simulink model "PTTransmCU"  (Simulink 10.3)
settings: Solver=ode45  StartTime=0.0  StopTime=inf  RelTol=1e-3  EnableMultiTasking=on
libraries: simulink x2, CarMaker4SL x1
(part 3 of 4)

== system PTTransmCU/CarMaker/IPG Vehicle/PowerTrain/TCU Example/PTTransmCU_In/CreateBus TCU ClutchIn5 ==
  In : Inport
  BusCreator : BusCreator  Inputs=7
  Demux : Demux  Outputs=7
      settings: DisplayOption=none
  Out : Outport  VectorParamsAs1DForOutWhenUnconnected=off
  wires:
  Demux/7 -> BusCreator/7  "TCU ClutchIn5 i_TrqIn2Out"
  Demux/6 -> BusCreator/6  "TCU ClutchIn5 Trq_out_trg"
  Demux/5 -> BusCreator/5  "TCU ClutchIn5 Trq_out"
  Demux/4 -> BusCreator/4  "TCU ClutchIn5 Trq_in"
  Demux/3 -> BusCreator/3  "TCU ClutchIn5 rotv_out_trg"
  Demux/2 -> BusCreator/2  "TCU ClutchIn5 rotv_out"
  Demux/1 -> BusCreator/1  "TCU ClutchIn5 rotv_in"
  BusCreator/1 -> Out/1
  In/1 -> Demux/1

== system PTTransmCU/CarMaker/IPG Vehicle/PowerTrain/TCU Example/PTTransmCU_In/CreateBus TCU ClutchIn6 ==
  In : Inport
  BusCreator : BusCreator  Inputs=7
  Demux : Demux  Outputs=7
      settings: DisplayOption=none
  Out : Outport  VectorParamsAs1DForOutWhenUnconnected=off
  wires:
  Demux/7 -> BusCreator/7  "TCU ClutchIn6 i_TrqIn2Out"
  Demux/6 -> BusCreator/6  "TCU ClutchIn6 Trq_out_trg"
  Demux/5 -> BusCreator/5  "TCU ClutchIn6 Trq_out"
  Demux/4 -> BusCreator/4  "TCU ClutchIn6 Trq_in"
  Demux/3 -> BusCreator/3  "TCU ClutchIn6 rotv_out_trg"
  Demux/2 -> BusCreator/2  "TCU ClutchIn6 rotv_out"
  Demux/1 -> BusCreator/1  "TCU ClutchIn6 rotv_in"
  BusCreator/1 -> Out/1
  In/1 -> Demux/1

== system PTTransmCU/CarMaker/IPG Vehicle/PowerTrain/TCU Example/PTTransmCU_In/CreateBus TCU ClutchIn7 ==
  In : Inport
  BusCreator : BusCreator  Inputs=7
  Demux : Demux  Outputs=7
      settings: DisplayOption=none
  Out : Outport  VectorParamsAs1DForOutWhenUnconnected=off
  wires:
  Demux/7 -> BusCreator/7  "TCU ClutchIn7 i_TrqIn2Out"
  Demux/6 -> BusCreator/6  "TCU ClutchIn7 Trq_out_trg"
  Demux/5 -> BusCreator/5  "TCU ClutchIn7 Trq_out"
  Demux/4 -> BusCreator/4  "TCU ClutchIn7 Trq_in"
  Demux/3 -> BusCreator/3  "TCU ClutchIn7 rotv_out_trg"
  Demux/2 -> BusCreator/2  "TCU ClutchIn7 rotv_out"
  Demux/1 -> BusCreator/1  "TCU ClutchIn7 rotv_in"
  BusCreator/1 -> Out/1
  In/1 -> Demux/1

== system PTTransmCU/CarMaker/IPG Vehicle/PowerTrain/TCU Example/PTTransmCU_In/CreateBus TCU ClutchIn8 ==
  In : Inport
  BusCreator : BusCreator  Inputs=7
  Demux : Demux  Outputs=7
      settings: DisplayOption=none
  Out : Outport  VectorParamsAs1DForOutWhenUnconnected=off
  wires:
  Demux/7 -> BusCreator/7  "TCU ClutchIn8 i_TrqIn2Out"
  Demux/6 -> BusCreator/6  "TCU ClutchIn8 Trq_out_trg"
  Demux/5 -> BusCreator/5  "TCU ClutchIn8 Trq_out"
  Demux/4 -> BusCreator/4  "TCU ClutchIn8 Trq_in"
  Demux/3 -> BusCreator/3  "TCU ClutchIn8 rotv_out_trg"
  Demux/2 -> BusCreator/2  "TCU ClutchIn8 rotv_out"
  Demux/1 -> BusCreator/1  "TCU ClutchIn8 rotv_in"
  BusCreator/1 -> Out/1
  In/1 -> Demux/1

== system PTTransmCU/CarMaker/IPG Vehicle/PowerTrain/TCU Example/PTTransmCU_In/CreateBus TCU ClutchIn9 ==
  In : Inport
  BusCreator : BusCreator  Inputs=7
  Demux : Demux  Outputs=7
      settings: DisplayOption=none
  Out : Outport  VectorParamsAs1DForOutWhenUnconnected=off
  wires:
  Demux/7 -> BusCreator/7  "TCU ClutchIn9 i_TrqIn2Out"
  Demux/6 -> BusCreator/6  "TCU ClutchIn9 Trq_out_trg"
  Demux/5 -> BusCreator/5  "TCU ClutchIn9 Trq_out"
  Demux/4 -> BusCreator/4  "TCU ClutchIn9 Trq_in"
  Demux/3 -> BusCreator/3  "TCU ClutchIn9 rotv_out_trg"
  Demux/2 -> BusCreator/2  "TCU ClutchIn9 rotv_out"
  Demux/1 -> BusCreator/1  "TCU ClutchIn9 rotv_in"
  BusCreator/1 -> Out/1
  In/1 -> Demux/1

== system PTTransmCU/CarMaker/IPG Vehicle/PowerTrain/TCU Example/PTTransmCU_In/CreateBus TCU ClutchOut0 ==
  In : Inport
  BusCreator : BusCreator  Inputs=1
  Demux : Demux  Outputs=1
      settings: DisplayOption=none
  Out : Outport  VectorParamsAs1DForOutWhenUnconnected=off
  wires:
  Demux/1 -> BusCreator/1  "TCU ClutchOut0 Pos"
  BusCreator/1 -> Out/1
  In/1 -> Demux/1

== system PTTransmCU/CarMaker/IPG Vehicle/PowerTrain/TCU Example/PTTransmCU_In/CreateBus TCU ClutchOut1 ==
  In : Inport
  BusCreator : BusCreator  Inputs=1
  Demux : Demux  Outputs=1
      settings: DisplayOption=none
  Out : Outport  VectorParamsAs1DForOutWhenUnconnected=off
  wires:
  Demux/1 -> BusCreator/1  "TCU ClutchOut1 Pos"
  BusCreator/1 -> Out/1
  In/1 -> Demux/1

== system PTTransmCU/CarMaker/IPG Vehicle/PowerTrain/TCU Example/PTTransmCU_In/CreateBus TCU ClutchOut10 ==
  In : Inport
  BusCreator : BusCreator  Inputs=1
  Demux : Demux  Outputs=1
      settings: DisplayOption=none
  Out : Outport  VectorParamsAs1DForOutWhenUnconnected=off
  wires:
  Demux/1 -> BusCreator/1  "TCU ClutchOut10 Pos"
  BusCreator/1 -> Out/1
  In/1 -> Demux/1

== system PTTransmCU/CarMaker/IPG Vehicle/PowerTrain/TCU Example/PTTransmCU_In/CreateBus TCU ClutchOut11 ==
  In : Inport
  BusCreator : BusCreator  Inputs=1
  Demux : Demux  Outputs=1
      settings: DisplayOption=none
  Out : Outport  VectorParamsAs1DForOutWhenUnconnected=off
  wires:
  Demux/1 -> BusCreator/1  "TCU ClutchOut11 Pos"
  BusCreator/1 -> Out/1
  In/1 -> Demux/1

== system PTTransmCU/CarMaker/IPG Vehicle/PowerTrain/TCU Example/PTTransmCU_In/CreateBus TCU ClutchOut2 ==
  In : Inport
  BusCreator : BusCreator  Inputs=1
  Demux : Demux  Outputs=1
      settings: DisplayOption=none
  Out : Outport  VectorParamsAs1DForOutWhenUnconnected=off
  wires:
  Demux/1 -> BusCreator/1  "TCU ClutchOut2 Pos"
  BusCreator/1 -> Out/1
  In/1 -> Demux/1

== system PTTransmCU/CarMaker/IPG Vehicle/PowerTrain/TCU Example/PTTransmCU_In/CreateBus TCU ClutchOut3 ==
  In : Inport
  BusCreator : BusCreator  Inputs=1
  Demux : Demux  Outputs=1
      settings: DisplayOption=none
  Out : Outport  VectorParamsAs1DForOutWhenUnconnected=off
  wires:
  Demux/1 -> BusCreator/1  "TCU ClutchOut3 Pos"
  BusCreator/1 -> Out/1
  In/1 -> Demux/1

== system PTTransmCU/CarMaker/IPG Vehicle/PowerTrain/TCU Example/PTTransmCU_In/CreateBus TCU ClutchOut4 ==
  In : Inport
  BusCreator : BusCreator  Inputs=1
  Demux : Demux  Outputs=1
      settings: DisplayOption=none
  Out : Outport  VectorParamsAs1DForOutWhenUnconnected=off
  wires:
  Demux/1 -> BusCreator/1  "TCU ClutchOut4 Pos"
  BusCreator/1 -> Out/1
  In/1 -> Demux/1

== system PTTransmCU/CarMaker/IPG Vehicle/PowerTrain/TCU Example/PTTransmCU_In/CreateBus TCU ClutchOut5 ==
  In : Inport
  BusCreator : BusCreator  Inputs=1
  Demux : Demux  Outputs=1
      settings: DisplayOption=none
  Out : Outport  VectorParamsAs1DForOutWhenUnconnected=off
  wires:
  Demux/1 -> BusCreator/1  "TCU ClutchOut5 Pos"
  BusCreator/1 -> Out/1
  In/1 -> Demux/1

== system PTTransmCU/CarMaker/IPG Vehicle/PowerTrain/TCU Example/PTTransmCU_In/CreateBus TCU ClutchOut6 ==
  In : Inport
  BusCreator : BusCreator  Inputs=1
  Demux : Demux  Outputs=1
      settings: DisplayOption=none
  Out : Outport  VectorParamsAs1DForOutWhenUnconnected=off
  wires:
  Demux/1 -> BusCreator/1  "TCU ClutchOut6 Pos"
  BusCreator/1 -> Out/1
  In/1 -> Demux/1

== system PTTransmCU/CarMaker/IPG Vehicle/PowerTrain/TCU Example/PTTransmCU_In/CreateBus TCU ClutchOut7 ==
  In : Inport
  BusCreator : BusCreator  Inputs=1
  Demux : Demux  Outputs=1
      settings: DisplayOption=none
  Out : Outport  VectorParamsAs1DForOutWhenUnconnected=off
  wires:
  Demux/1 -> BusCreator/1  "TCU ClutchOut7 Pos"
  BusCreator/1 -> Out/1
  In/1 -> Demux/1

== system PTTransmCU/CarMaker/IPG Vehicle/PowerTrain/TCU Example/PTTransmCU_In/CreateBus TCU ClutchOut8 ==
  In : Inport
  BusCreator : BusCreator  Inputs=1
  Demux : Demux  Outputs=1
      settings: DisplayOption=none
  Out : Outport  VectorParamsAs1DForOutWhenUnconnected=off
  wires:
  Demux/1 -> BusCreator/1  "TCU ClutchOut8 Pos"
  BusCreator/1 -> Out/1
  In/1 -> Demux/1

== system PTTransmCU/CarMaker/IPG Vehicle/PowerTrain/TCU Example/PTTransmCU_In/CreateBus TCU ClutchOut9 ==
  In : Inport
  BusCreator : BusCreator  Inputs=1
  Demux : Demux  Outputs=1
      settings: DisplayOption=none
  Out : Outport  VectorParamsAs1DForOutWhenUnconnected=off
  wires:
  Demux/1 -> BusCreator/1  "TCU ClutchOut9 Pos"
  BusCreator/1 -> Out/1
  In/1 -> Demux/1

== system PTTransmCU/CarMaker/IPG Vehicle/PowerTrain/TCU Example/PTTransmCU_In/CreateBus TCU GearboxIn0 ==
  In : Inport
  BusCreator : BusCreator  Inputs=23
  Demux : Demux  Outputs=23
      settings: DisplayOption=none
  Out : Outport  VectorParamsAs1DForOutWhenUnconnected=off
  wires:
  Demux/23 -> BusCreator/23  "TCU GearboxIn0 Clutch_dis i_TrqIn2Out"
  Demux/22 -> BusCreator/22  "TCU GearboxIn0 Clutch_dis Trq_out_trg"
  Demux/21 -> BusCreator/21  "TCU GearboxIn0 Clutch_dis Trq_out"
  Demux/20 -> BusCreator/20  "TCU GearboxIn0 Clutch_dis Trq_in"
  Demux/19 -> BusCreator/19  "TCU GearboxIn0 Clutch_dis rotv_out_trg"
  Demux/18 -> BusCreator/18  "TCU GearboxIn0 Clutch_dis rotv_out"
  Demux/17 -> BusCreator/17  "TCU GearboxIn0 Clutch_dis rotv_in"
  Demux/16 -> BusCreator/16  "TCU GearboxIn0 Clutch i_TrqIn2Out"
  Demux/15 -> BusCreator/15  "TCU GearboxIn0 Clutch Trq_out_trg"
  Demux/14 -> BusCreator/14  "TCU GearboxIn0 Clutch Trq_out"
  Demux/13 -> BusCreator/13  "TCU GearboxIn0 Clutch Trq_in"
  Demux/12 -> BusCreator/12  "TCU GearboxIn0 Clutch rotv_out_trg"
  Demux/11 -> BusCreator/11  "TCU GearboxIn0 Clutch rotv_out"
  Demux/10 -> BusCreator/10  "TCU GearboxIn0 Clutch rotv_in"
  Demux/9 -> BusCreator/9  "TCU GearboxIn0 Trq_out_trg"
  Demux/8 -> BusCreator/8  "TCU GearboxIn0 Trq_out"
  Demux/7 -> BusCreator/7  "TCU GearboxIn0 Trq_in"
  Demux/6 -> BusCreator/6  "TCU GearboxIn0 rotv_out"
  Demux/5 -> BusCreator/5  "TCU GearboxIn0 rotv_in_trg"
  Demux/4 -> BusCreator/4  "TCU GearboxIn0 rotv_in"
  Demux/3 -> BusCreator/3  "TCU GearboxIn0 i"
  Demux/2 -> BusCreator/2  "TCU GearboxIn0 GearNo_dis"
  Demux/1 -> BusCreator/1  "TCU GearboxIn0 GearNo"
  BusCreator/1 -> Out/1
  In/1 -> Demux/1

== system PTTransmCU/CarMaker/IPG Vehicle/PowerTrain/TCU Example/PTTransmCU_In/CreateBus TCU GearboxIn1 ==
  In : Inport
  BusCreator : BusCreator  Inputs=23
  Demux : Demux  Outputs=23
      settings: DisplayOption=none
  Out : Outport  VectorParamsAs1DForOutWhenUnconnected=off
  wires:
  Demux/23 -> BusCreator/23  "TCU GearboxIn1 Clutch_dis i_TrqIn2Out"
  Demux/22 -> BusCreator/22  "TCU GearboxIn1 Clutch_dis Trq_out_trg"
  Demux/21 -> BusCreator/21  "TCU GearboxIn1 Clutch_dis Trq_out"
  Demux/20 -> BusCreator/20  "TCU GearboxIn1 Clutch_dis Trq_in"
  Demux/19 -> BusCreator/19  "TCU GearboxIn1 Clutch_dis rotv_out_trg"
  Demux/18 -> BusCreator/18  "TCU GearboxIn1 Clutch_dis rotv_out"
  Demux/17 -> BusCreator/17  "TCU GearboxIn1 Clutch_dis rotv_in"
  Demux/16 -> BusCreator/16  "TCU GearboxIn1 Clutch i_TrqIn2Out"
  Demux/15 -> BusCreator/15  "TCU GearboxIn1 Clutch Trq_out_trg"
  Demux/14 -> BusCreator/14  "TCU GearboxIn1 Clutch Trq_out"
  Demux/13 -> BusCreator/13  "TCU GearboxIn1 Clutch Trq_in"
  Demux/12 -> BusCreator/12  "TCU GearboxIn1 Clutch rotv_out_trg"
  Demux/11 -> BusCreator/11  "TCU GearboxIn1 Clutch rotv_out"
  Demux/10 -> BusCreator/10  "TCU GearboxIn1 Clutch rotv_in"
  Demux/9 -> BusCreator/9  "TCU GearboxIn1 Trq_out_trg"
  Demux/8 -> BusCreator/8  "TCU GearboxIn1 Trq_out"
  Demux/7 -> BusCreator/7  "TCU GearboxIn1 Trq_in"
  Demux/6 -> BusCreator/6  "TCU GearboxIn1 rotv_out"
  Demux/5 -> BusCreator/5  "TCU GearboxIn1 rotv_in_trg"
  Demux/4 -> BusCreator/4  "TCU GearboxIn1 rotv_in"
  Demux/3 -> BusCreator/3  "TCU GearboxIn1 i"
  Demux/2 -> BusCreator/2  "TCU GearboxIn1 GearNo_dis"
  Demux/1 -> BusCreator/1  "TCU GearboxIn1 GearNo"
  BusCreator/1 -> Out/1
  In/1 -> Demux/1

== system PTTransmCU/CarMaker/IPG Vehicle/PowerTrain/TCU Example/PTTransmCU_In/CreateBus TCU GearboxIn10 ==
  In : Inport
  BusCreator : BusCreator  Inputs=23
  Demux : Demux  Outputs=23
      settings: DisplayOption=none
  Out : Outport  VectorParamsAs1DForOutWhenUnconnected=off
  wires:
  Demux/23 -> BusCreator/23  "TCU GearboxIn10 Clutch_dis i_TrqIn2Out"
  Demux/22 -> BusCreator/22  "TCU GearboxIn10 Clutch_dis Trq_out_trg"
  Demux/21 -> BusCreator/21  "TCU GearboxIn10 Clutch_dis Trq_out"
  Demux/20 -> BusCreator/20  "TCU GearboxIn10 Clutch_dis Trq_in"
  Demux/19 -> BusCreator/19  "TCU GearboxIn10 Clutch_dis rotv_out_trg"
  Demux/18 -> BusCreator/18  "TCU GearboxIn10 Clutch_dis rotv_out"
  Demux/17 -> BusCreator/17  "TCU GearboxIn10 Clutch_dis rotv_in"
  Demux/16 -> BusCreator/16  "TCU GearboxIn10 Clutch i_TrqIn2Out"
  Demux/15 -> BusCreator/15  "TCU GearboxIn10 Clutch Trq_out_trg"
  Demux/14 -> BusCreator/14  "TCU GearboxIn10 Clutch Trq_out"
  Demux/13 -> BusCreator/13  "TCU GearboxIn10 Clutch Trq_in"
  Demux/12 -> BusCreator/12  "TCU GearboxIn10 Clutch rotv_out_trg"
  Demux/11 -> BusCreator/11  "TCU GearboxIn10 Clutch rotv_out"
  Demux/10 -> BusCreator/10  "TCU GearboxIn10 Clutch rotv_in"
  Demux/9 -> BusCreator/9  "TCU GearboxIn10 Trq_out_trg"
  Demux/8 -> BusCreator/8  "TCU GearboxIn10 Trq_out"
  Demux/7 -> BusCreator/7  "TCU GearboxIn10 Trq_in"
  Demux/6 -> BusCreator/6  "TCU GearboxIn10 rotv_out"
  Demux/5 -> BusCreator/5  "TCU GearboxIn10 rotv_in_trg"
  Demux/4 -> BusCreator/4  "TCU GearboxIn10 rotv_in"
  Demux/3 -> BusCreator/3  "TCU GearboxIn10 i"
  Demux/2 -> BusCreator/2  "TCU GearboxIn10 GearNo_dis"
  Demux/1 -> BusCreator/1  "TCU GearboxIn10 GearNo"
  BusCreator/1 -> Out/1
  In/1 -> Demux/1

== system PTTransmCU/CarMaker/IPG Vehicle/PowerTrain/TCU Example/PTTransmCU_In/CreateBus TCU GearboxIn11 ==
  In : Inport
  BusCreator : BusCreator  Inputs=23
  Demux : Demux  Outputs=23
      settings: DisplayOption=none
  Out : Outport  VectorParamsAs1DForOutWhenUnconnected=off
  wires:
  Demux/23 -> BusCreator/23  "TCU GearboxIn11 Clutch_dis i_TrqIn2Out"
  Demux/22 -> BusCreator/22  "TCU GearboxIn11 Clutch_dis Trq_out_trg"
  Demux/21 -> BusCreator/21  "TCU GearboxIn11 Clutch_dis Trq_out"
  Demux/20 -> BusCreator/20  "TCU GearboxIn11 Clutch_dis Trq_in"
  Demux/19 -> BusCreator/19  "TCU GearboxIn11 Clutch_dis rotv_out_trg"
  Demux/18 -> BusCreator/18  "TCU GearboxIn11 Clutch_dis rotv_out"
  Demux/17 -> BusCreator/17  "TCU GearboxIn11 Clutch_dis rotv_in"
  Demux/16 -> BusCreator/16  "TCU GearboxIn11 Clutch i_TrqIn2Out"
  Demux/15 -> BusCreator/15  "TCU GearboxIn11 Clutch Trq_out_trg"
  Demux/14 -> BusCreator/14  "TCU GearboxIn11 Clutch Trq_out"
  Demux/13 -> BusCreator/13  "TCU GearboxIn11 Clutch Trq_in"
  Demux/12 -> BusCreator/12  "TCU GearboxIn11 Clutch rotv_out_trg"
  Demux/11 -> BusCreator/11  "TCU GearboxIn11 Clutch rotv_out"
  Demux/10 -> BusCreator/10  "TCU GearboxIn11 Clutch rotv_in"
  Demux/9 -> BusCreator/9  "TCU GearboxIn11 Trq_out_trg"
  Demux/8 -> BusCreator/8  "TCU GearboxIn11 Trq_out"
  Demux/7 -> BusCreator/7  "TCU GearboxIn11 Trq_in"
  Demux/6 -> BusCreator/6  "TCU GearboxIn11 rotv_out"
  Demux/5 -> BusCreator/5  "TCU GearboxIn11 rotv_in_trg"
  Demux/4 -> BusCreator/4  "TCU GearboxIn11 rotv_in"
  Demux/3 -> BusCreator/3  "TCU GearboxIn11 i"
  Demux/2 -> BusCreator/2  "TCU GearboxIn11 GearNo_dis"
  Demux/1 -> BusCreator/1  "TCU GearboxIn11 GearNo"
  BusCreator/1 -> Out/1
  In/1 -> Demux/1

== system PTTransmCU/CarMaker/IPG Vehicle/PowerTrain/TCU Example/PTTransmCU_In/CreateBus TCU GearboxIn2 ==
  In : Inport
  BusCreator : BusCreator  Inputs=23
  Demux : Demux  Outputs=23
      settings: DisplayOption=none
  Out : Outport  VectorParamsAs1DForOutWhenUnconnected=off
  wires:
  Demux/23 -> BusCreator/23  "TCU GearboxIn2 Clutch_dis i_TrqIn2Out"
  Demux/22 -> BusCreator/22  "TCU GearboxIn2 Clutch_dis Trq_out_trg"
  Demux/21 -> BusCreator/21  "TCU GearboxIn2 Clutch_dis Trq_out"
  Demux/20 -> BusCreator/20  "TCU GearboxIn2 Clutch_dis Trq_in"
  Demux/19 -> BusCreator/19  "TCU GearboxIn2 Clutch_dis rotv_out_trg"
  Demux/18 -> BusCreator/18  "TCU GearboxIn2 Clutch_dis rotv_out"
  Demux/17 -> BusCreator/17  "TCU GearboxIn2 Clutch_dis rotv_in"
  Demux/16 -> BusCreator/16  "TCU GearboxIn2 Clutch i_TrqIn2Out"
  Demux/15 -> BusCreator/15  "TCU GearboxIn2 Clutch Trq_out_trg"
  Demux/14 -> BusCreator/14  "TCU GearboxIn2 Clutch Trq_out"
  Demux/13 -> BusCreator/13  "TCU GearboxIn2 Clutch Trq_in"
  Demux/12 -> BusCreator/12  "TCU GearboxIn2 Clutch rotv_out_trg"
  Demux/11 -> BusCreator/11  "TCU GearboxIn2 Clutch rotv_out"
  Demux/10 -> BusCreator/10  "TCU GearboxIn2 Clutch rotv_in"
  Demux/9 -> BusCreator/9  "TCU GearboxIn2 Trq_out_trg"
  Demux/8 -> BusCreator/8  "TCU GearboxIn2 Trq_out"
  Demux/7 -> BusCreator/7  "TCU GearboxIn2 Trq_in"
  Demux/6 -> BusCreator/6  "TCU GearboxIn2 rotv_out"
  Demux/5 -> BusCreator/5  "TCU GearboxIn2 rotv_in_trg"
  Demux/4 -> BusCreator/4  "TCU GearboxIn2 rotv_in"
  Demux/3 -> BusCreator/3  "TCU GearboxIn2 i"
  Demux/2 -> BusCreator/2  "TCU GearboxIn2 GearNo_dis"
  Demux/1 -> BusCreator/1  "TCU GearboxIn2 GearNo"
  BusCreator/1 -> Out/1
  In/1 -> Demux/1

== system PTTransmCU/CarMaker/IPG Vehicle/PowerTrain/TCU Example/PTTransmCU_In/CreateBus TCU GearboxIn3 ==
  In : Inport
  BusCreator : BusCreator  Inputs=23
  Demux : Demux  Outputs=23
      settings: DisplayOption=none
  Out : Outport  VectorParamsAs1DForOutWhenUnconnected=off
  wires:
  Demux/23 -> BusCreator/23  "TCU GearboxIn3 Clutch_dis i_TrqIn2Out"
  Demux/22 -> BusCreator/22  "TCU GearboxIn3 Clutch_dis Trq_out_trg"
  Demux/21 -> BusCreator/21  "TCU GearboxIn3 Clutch_dis Trq_out"
  Demux/20 -> BusCreator/20  "TCU GearboxIn3 Clutch_dis Trq_in"
  Demux/19 -> BusCreator/19  "TCU GearboxIn3 Clutch_dis rotv_out_trg"
  Demux/18 -> BusCreator/18  "TCU GearboxIn3 Clutch_dis rotv_out"
  Demux/17 -> BusCreator/17  "TCU GearboxIn3 Clutch_dis rotv_in"
  Demux/16 -> BusCreator/16  "TCU GearboxIn3 Clutch i_TrqIn2Out"
  Demux/15 -> BusCreator/15  "TCU GearboxIn3 Clutch Trq_out_trg"
  Demux/14 -> BusCreator/14  "TCU GearboxIn3 Clutch Trq_out"
  Demux/13 -> BusCreator/13  "TCU GearboxIn3 Clutch Trq_in"
  Demux/12 -> BusCreator/12  "TCU GearboxIn3 Clutch rotv_out_trg"
  Demux/11 -> BusCreator/11  "TCU GearboxIn3 Clutch rotv_out"
  Demux/10 -> BusCreator/10  "TCU GearboxIn3 Clutch rotv_in"
  Demux/9 -> BusCreator/9  "TCU GearboxIn3 Trq_out_trg"
  Demux/8 -> BusCreator/8  "TCU GearboxIn3 Trq_out"
  Demux/7 -> BusCreator/7  "TCU GearboxIn3 Trq_in"
  Demux/6 -> BusCreator/6  "TCU GearboxIn3 rotv_out"
  Demux/5 -> BusCreator/5  "TCU GearboxIn3 rotv_in_trg"
  Demux/4 -> BusCreator/4  "TCU GearboxIn3 rotv_in"
  Demux/3 -> BusCreator/3  "TCU GearboxIn3 i"
  Demux/2 -> BusCreator/2  "TCU GearboxIn3 GearNo_dis"
  Demux/1 -> BusCreator/1  "TCU GearboxIn3 GearNo"
  BusCreator/1 -> Out/1
  In/1 -> Demux/1

== system PTTransmCU/CarMaker/IPG Vehicle/PowerTrain/TCU Example/PTTransmCU_In/CreateBus TCU GearboxIn4 ==
  In : Inport
  BusCreator : BusCreator  Inputs=23
  Demux : Demux  Outputs=23
      settings: DisplayOption=none
  Out : Outport  VectorParamsAs1DForOutWhenUnconnected=off
  wires:
  Demux/23 -> BusCreator/23  "TCU GearboxIn4 Clutch_dis i_TrqIn2Out"
  Demux/22 -> BusCreator/22  "TCU GearboxIn4 Clutch_dis Trq_out_trg"
  Demux/21 -> BusCreator/21  "TCU GearboxIn4 Clutch_dis Trq_out"
  Demux/20 -> BusCreator/20  "TCU GearboxIn4 Clutch_dis Trq_in"
  Demux/19 -> BusCreator/19  "TCU GearboxIn4 Clutch_dis rotv_out_trg"
  Demux/18 -> BusCreator/18  "TCU GearboxIn4 Clutch_dis rotv_out"
  Demux/17 -> BusCreator/17  "TCU GearboxIn4 Clutch_dis rotv_in"
  Demux/16 -> BusCreator/16  "TCU GearboxIn4 Clutch i_TrqIn2Out"
  Demux/15 -> BusCreator/15  "TCU GearboxIn4 Clutch Trq_out_trg"
  Demux/14 -> BusCreator/14  "TCU GearboxIn4 Clutch Trq_out"
  Demux/13 -> BusCreator/13  "TCU GearboxIn4 Clutch Trq_in"
  Demux/12 -> BusCreator/12  "TCU GearboxIn4 Clutch rotv_out_trg"
  Demux/11 -> BusCreator/11  "TCU GearboxIn4 Clutch rotv_out"
  Demux/10 -> BusCreator/10  "TCU GearboxIn4 Clutch rotv_in"
  Demux/9 -> BusCreator/9  "TCU GearboxIn4 Trq_out_trg"
  Demux/8 -> BusCreator/8  "TCU GearboxIn4 Trq_out"
  Demux/7 -> BusCreator/7  "TCU GearboxIn4 Trq_in"
  Demux/6 -> BusCreator/6  "TCU GearboxIn4 rotv_out"
  Demux/5 -> BusCreator/5  "TCU GearboxIn4 rotv_in_trg"
  Demux/4 -> BusCreator/4  "TCU GearboxIn4 rotv_in"
  Demux/3 -> BusCreator/3  "TCU GearboxIn4 i"
  Demux/2 -> BusCreator/2  "TCU GearboxIn4 GearNo_dis"
  Demux/1 -> BusCreator/1  "TCU GearboxIn4 GearNo"
  BusCreator/1 -> Out/1
  In/1 -> Demux/1

== system PTTransmCU/CarMaker/IPG Vehicle/PowerTrain/TCU Example/PTTransmCU_In/CreateBus TCU GearboxIn5 ==
  In : Inport
  BusCreator : BusCreator  Inputs=23
  Demux : Demux  Outputs=23
      settings: DisplayOption=none
  Out : Outport  VectorParamsAs1DForOutWhenUnconnected=off
  wires:
  Demux/23 -> BusCreator/23  "TCU GearboxIn5 Clutch_dis i_TrqIn2Out"
  Demux/22 -> BusCreator/22  "TCU GearboxIn5 Clutch_dis Trq_out_trg"
  Demux/21 -> BusCreator/21  "TCU GearboxIn5 Clutch_dis Trq_out"
  Demux/20 -> BusCreator/20  "TCU GearboxIn5 Clutch_dis Trq_in"
  Demux/19 -> BusCreator/19  "TCU GearboxIn5 Clutch_dis rotv_out_trg"
  Demux/18 -> BusCreator/18  "TCU GearboxIn5 Clutch_dis rotv_out"
  Demux/17 -> BusCreator/17  "TCU GearboxIn5 Clutch_dis rotv_in"
  Demux/16 -> BusCreator/16  "TCU GearboxIn5 Clutch i_TrqIn2Out"
  Demux/15 -> BusCreator/15  "TCU GearboxIn5 Clutch Trq_out_trg"
  Demux/14 -> BusCreator/14  "TCU GearboxIn5 Clutch Trq_out"
  Demux/13 -> BusCreator/13  "TCU GearboxIn5 Clutch Trq_in"
  Demux/12 -> BusCreator/12  "TCU GearboxIn5 Clutch rotv_out_trg"
  Demux/11 -> BusCreator/11  "TCU GearboxIn5 Clutch rotv_out"
  Demux/10 -> BusCreator/10  "TCU GearboxIn5 Clutch rotv_in"
  Demux/9 -> BusCreator/9  "TCU GearboxIn5 Trq_out_trg"
  Demux/8 -> BusCreator/8  "TCU GearboxIn5 Trq_out"
  Demux/7 -> BusCreator/7  "TCU GearboxIn5 Trq_in"
  Demux/6 -> BusCreator/6  "TCU GearboxIn5 rotv_out"
  Demux/5 -> BusCreator/5  "TCU GearboxIn5 rotv_in_trg"
  Demux/4 -> BusCreator/4  "TCU GearboxIn5 rotv_in"
  Demux/3 -> BusCreator/3  "TCU GearboxIn5 i"
  Demux/2 -> BusCreator/2  "TCU GearboxIn5 GearNo_dis"
  Demux/1 -> BusCreator/1  "TCU GearboxIn5 GearNo"
  BusCreator/1 -> Out/1
  In/1 -> Demux/1

== system PTTransmCU/CarMaker/IPG Vehicle/PowerTrain/TCU Example/PTTransmCU_In/CreateBus TCU GearboxIn6 ==
  In : Inport
  BusCreator : BusCreator  Inputs=23
  Demux : Demux  Outputs=23
      settings: DisplayOption=none
  Out : Outport  VectorParamsAs1DForOutWhenUnconnected=off
  wires:
  Demux/23 -> BusCreator/23  "TCU GearboxIn6 Clutch_dis i_TrqIn2Out"
  Demux/22 -> BusCreator/22  "TCU GearboxIn6 Clutch_dis Trq_out_trg"
  Demux/21 -> BusCreator/21  "TCU GearboxIn6 Clutch_dis Trq_out"
  Demux/20 -> BusCreator/20  "TCU GearboxIn6 Clutch_dis Trq_in"
  Demux/19 -> BusCreator/19  "TCU GearboxIn6 Clutch_dis rotv_out_trg"
  Demux/18 -> BusCreator/18  "TCU GearboxIn6 Clutch_dis rotv_out"
  Demux/17 -> BusCreator/17  "TCU GearboxIn6 Clutch_dis rotv_in"
  Demux/16 -> BusCreator/16  "TCU GearboxIn6 Clutch i_TrqIn2Out"
  Demux/15 -> BusCreator/15  "TCU GearboxIn6 Clutch Trq_out_trg"
  Demux/14 -> BusCreator/14  "TCU GearboxIn6 Clutch Trq_out"
  Demux/13 -> BusCreator/13  "TCU GearboxIn6 Clutch Trq_in"
  Demux/12 -> BusCreator/12  "TCU GearboxIn6 Clutch rotv_out_trg"
  Demux/11 -> BusCreator/11  "TCU GearboxIn6 Clutch rotv_out"
  Demux/10 -> BusCreator/10  "TCU GearboxIn6 Clutch rotv_in"
  Demux/9 -> BusCreator/9  "TCU GearboxIn6 Trq_out_trg"
  Demux/8 -> BusCreator/8  "TCU GearboxIn6 Trq_out"
  Demux/7 -> BusCreator/7  "TCU GearboxIn6 Trq_in"
  Demux/6 -> BusCreator/6  "TCU GearboxIn6 rotv_out"
  Demux/5 -> BusCreator/5  "TCU GearboxIn6 rotv_in_trg"
  Demux/4 -> BusCreator/4  "TCU GearboxIn6 rotv_in"
  Demux/3 -> BusCreator/3  "TCU GearboxIn6 i"
  Demux/2 -> BusCreator/2  "TCU GearboxIn6 GearNo_dis"
  Demux/1 -> BusCreator/1  "TCU GearboxIn6 GearNo"
  BusCreator/1 -> Out/1
  In/1 -> Demux/1

== system PTTransmCU/CarMaker/IPG Vehicle/PowerTrain/TCU Example/PTTransmCU_In/CreateBus TCU GearboxIn7 ==
  In : Inport
  BusCreator : BusCreator  Inputs=23
  Demux : Demux  Outputs=23
      settings: DisplayOption=none
  Out : Outport  VectorParamsAs1DForOutWhenUnconnected=off
  wires:
  Demux/23 -> BusCreator/23  "TCU GearboxIn7 Clutch_dis i_TrqIn2Out"
  Demux/22 -> BusCreator/22  "TCU GearboxIn7 Clutch_dis Trq_out_trg"
  Demux/21 -> BusCreator/21  "TCU GearboxIn7 Clutch_dis Trq_out"
  Demux/20 -> BusCreator/20  "TCU GearboxIn7 Clutch_dis Trq_in"
  Demux/19 -> BusCreator/19  "TCU GearboxIn7 Clutch_dis rotv_out_trg"
  Demux/18 -> BusCreator/18  "TCU GearboxIn7 Clutch_dis rotv_out"
  Demux/17 -> BusCreator/17  "TCU GearboxIn7 Clutch_dis rotv_in"
  Demux/16 -> BusCreator/16  "TCU GearboxIn7 Clutch i_TrqIn2Out"
  Demux/15 -> BusCreator/15  "TCU GearboxIn7 Clutch Trq_out_trg"
  Demux/14 -> BusCreator/14  "TCU GearboxIn7 Clutch Trq_out"
  Demux/13 -> BusCreator/13  "TCU GearboxIn7 Clutch Trq_in"
  Demux/12 -> BusCreator/12  "TCU GearboxIn7 Clutch rotv_out_trg"
  Demux/11 -> BusCreator/11  "TCU GearboxIn7 Clutch rotv_out"
  Demux/10 -> BusCreator/10  "TCU GearboxIn7 Clutch rotv_in"
  Demux/9 -> BusCreator/9  "TCU GearboxIn7 Trq_out_trg"
  Demux/8 -> BusCreator/8  "TCU GearboxIn7 Trq_out"
  Demux/7 -> BusCreator/7  "TCU GearboxIn7 Trq_in"
  Demux/6 -> BusCreator/6  "TCU GearboxIn7 rotv_out"
  Demux/5 -> BusCreator/5  "TCU GearboxIn7 rotv_in_trg"
  Demux/4 -> BusCreator/4  "TCU GearboxIn7 rotv_in"
  Demux/3 -> BusCreator/3  "TCU GearboxIn7 i"
  Demux/2 -> BusCreator/2  "TCU GearboxIn7 GearNo_dis"
  Demux/1 -> BusCreator/1  "TCU GearboxIn7 GearNo"
  BusCreator/1 -> Out/1
  In/1 -> Demux/1

== system PTTransmCU/CarMaker/IPG Vehicle/PowerTrain/TCU Example/PTTransmCU_In/CreateBus TCU GearboxIn8 ==
  In : Inport
  BusCreator : BusCreator  Inputs=23
  Demux : Demux  Outputs=23
      settings: DisplayOption=none
  Out : Outport  VectorParamsAs1DForOutWhenUnconnected=off
  wires:
  Demux/23 -> BusCreator/23  "TCU GearboxIn8 Clutch_dis i_TrqIn2Out"
  Demux/22 -> BusCreator/22  "TCU GearboxIn8 Clutch_dis Trq_out_trg"
  Demux/21 -> BusCreator/21  "TCU GearboxIn8 Clutch_dis Trq_out"
  Demux/20 -> BusCreator/20  "TCU GearboxIn8 Clutch_dis Trq_in"
  Demux/19 -> BusCreator/19  "TCU GearboxIn8 Clutch_dis rotv_out_trg"
  Demux/18 -> BusCreator/18  "TCU GearboxIn8 Clutch_dis rotv_out"
  Demux/17 -> BusCreator/17  "TCU GearboxIn8 Clutch_dis rotv_in"
  Demux/16 -> BusCreator/16  "TCU GearboxIn8 Clutch i_TrqIn2Out"
  Demux/15 -> BusCreator/15  "TCU GearboxIn8 Clutch Trq_out_trg"
  Demux/14 -> BusCreator/14  "TCU GearboxIn8 Clutch Trq_out"
  Demux/13 -> BusCreator/13  "TCU GearboxIn8 Clutch Trq_in"
  Demux/12 -> BusCreator/12  "TCU GearboxIn8 Clutch rotv_out_trg"
  Demux/11 -> BusCreator/11  "TCU GearboxIn8 Clutch rotv_out"
  Demux/10 -> BusCreator/10  "TCU GearboxIn8 Clutch rotv_in"
  Demux/9 -> BusCreator/9  "TCU GearboxIn8 Trq_out_trg"
  Demux/8 -> BusCreator/8  "TCU GearboxIn8 Trq_out"
  Demux/7 -> BusCreator/7  "TCU GearboxIn8 Trq_in"
  Demux/6 -> BusCreator/6  "TCU GearboxIn8 rotv_out"
  Demux/5 -> BusCreator/5  "TCU GearboxIn8 rotv_in_trg"
  Demux/4 -> BusCreator/4  "TCU GearboxIn8 rotv_in"
  Demux/3 -> BusCreator/3  "TCU GearboxIn8 i"
  Demux/2 -> BusCreator/2  "TCU GearboxIn8 GearNo_dis"
  Demux/1 -> BusCreator/1  "TCU GearboxIn8 GearNo"
  BusCreator/1 -> Out/1
  In/1 -> Demux/1

== system PTTransmCU/CarMaker/IPG Vehicle/PowerTrain/TCU Example/PTTransmCU_In/CreateBus TCU GearboxIn9 ==
  In : Inport
  BusCreator : BusCreator  Inputs=23
  Demux : Demux  Outputs=23
      settings: DisplayOption=none
  Out : Outport  VectorParamsAs1DForOutWhenUnconnected=off
  wires:
  Demux/23 -> BusCreator/23  "TCU GearboxIn9 Clutch_dis i_TrqIn2Out"
  Demux/22 -> BusCreator/22  "TCU GearboxIn9 Clutch_dis Trq_out_trg"
  Demux/21 -> BusCreator/21  "TCU GearboxIn9 Clutch_dis Trq_out"
  Demux/20 -> BusCreator/20  "TCU GearboxIn9 Clutch_dis Trq_in"
  Demux/19 -> BusCreator/19  "TCU GearboxIn9 Clutch_dis rotv_out_trg"
  Demux/18 -> BusCreator/18  "TCU GearboxIn9 Clutch_dis rotv_out"
  Demux/17 -> BusCreator/17  "TCU GearboxIn9 Clutch_dis rotv_in"
  Demux/16 -> BusCreator/16  "TCU GearboxIn9 Clutch i_TrqIn2Out"
  Demux/15 -> BusCreator/15  "TCU GearboxIn9 Clutch Trq_out_trg"
  Demux/14 -> BusCreator/14  "TCU GearboxIn9 Clutch Trq_out"
  Demux/13 -> BusCreator/13  "TCU GearboxIn9 Clutch Trq_in"
  Demux/12 -> BusCreator/12  "TCU GearboxIn9 Clutch rotv_out_trg"
  Demux/11 -> BusCreator/11  "TCU GearboxIn9 Clutch rotv_out"
  Demux/10 -> BusCreator/10  "TCU GearboxIn9 Clutch rotv_in"
  Demux/9 -> BusCreator/9  "TCU GearboxIn9 Trq_out_trg"
  Demux/8 -> BusCreator/8  "TCU GearboxIn9 Trq_out"
  Demux/7 -> BusCreator/7  "TCU GearboxIn9 Trq_in"
  Demux/6 -> BusCreator/6  "TCU GearboxIn9 rotv_out"
  Demux/5 -> BusCreator/5  "TCU GearboxIn9 rotv_in_trg"
  Demux/4 -> BusCreator/4  "TCU GearboxIn9 rotv_in"
  Demux/3 -> BusCreator/3  "TCU GearboxIn9 i"
  Demux/2 -> BusCreator/2  "TCU GearboxIn9 GearNo_dis"
  Demux/1 -> BusCreator/1  "TCU GearboxIn9 GearNo"
  BusCreator/1 -> Out/1
  In/1 -> Demux/1

== system PTTransmCU/CarMaker/IPG Vehicle/PowerTrain/TCU Example/PTTransmCU_In/CreateBus TCU GearboxOut0 ==
  In : Inport
  BusCreator : BusCreator  Inputs=6
  Demux : Demux  Outputs=6
      settings: DisplayOption=none
  Out : Outport  VectorParamsAs1DForOutWhenUnconnected=off
  wires:
  Demux/6 -> BusCreator/6  "TCU GearboxOut0 Clutch_dis Pos"
  Demux/5 -> BusCreator/5  "TCU GearboxOut0 Clutch Pos"
  Demux/4 -> BusCreator/4  "TCU GearboxOut0 i_trg"
  Demux/3 -> BusCreator/3  "TCU GearboxOut0 set_ParkBrake"
  Demux/2 -> BusCreator/2  "TCU GearboxOut0 GearNoTrg_dis"
  Demux/1 -> BusCreator/1  "TCU GearboxOut0 GearNoTrg"
  BusCreator/1 -> Out/1
  In/1 -> Demux/1

== system PTTransmCU/CarMaker/IPG Vehicle/PowerTrain/TCU Example/PTTransmCU_In/CreateBus TCU GearboxOut1 ==
  In : Inport
  BusCreator : BusCreator  Inputs=6
  Demux : Demux  Outputs=6
      settings: DisplayOption=none
  Out : Outport  VectorParamsAs1DForOutWhenUnconnected=off
  wires:
  Demux/6 -> BusCreator/6  "TCU GearboxOut1 Clutch_dis Pos"
  Demux/5 -> BusCreator/5  "TCU GearboxOut1 Clutch Pos"
  Demux/4 -> BusCreator/4  "TCU GearboxOut1 i_trg"
  Demux/3 -> BusCreator/3  "TCU GearboxOut1 set_ParkBrake"
  Demux/2 -> BusCreator/2  "TCU GearboxOut1 GearNoTrg_dis"
  Demux/1 -> BusCreator/1  "TCU GearboxOut1 GearNoTrg"
  BusCreator/1 -> Out/1
  In/1 -> Demux/1

== system PTTransmCU/CarMaker/IPG Vehicle/PowerTrain/TCU Example/PTTransmCU_In/CreateBus TCU GearboxOut10 ==
  In : Inport
  BusCreator : BusCreator  Inputs=6
  Demux : Demux  Outputs=6
      settings: DisplayOption=none
  Out : Outport  VectorParamsAs1DForOutWhenUnconnected=off
  wires:
  Demux/6 -> BusCreator/6  "TCU GearboxOut10 Clutch_dis Pos"
  Demux/5 -> BusCreator/5  "TCU GearboxOut10 Clutch Pos"
  Demux/4 -> BusCreator/4  "TCU GearboxOut10 i_trg"
  Demux/3 -> BusCreator/3  "TCU GearboxOut10 set_ParkBrake"
  Demux/2 -> BusCreator/2  "TCU GearboxOut10 GearNoTrg_dis"
  Demux/1 -> BusCreator/1  "TCU GearboxOut10 GearNoTrg"
  BusCreator/1 -> Out/1
  In/1 -> Demux/1

== system PTTransmCU/CarMaker/IPG Vehicle/PowerTrain/TCU Example/PTTransmCU_In/CreateBus TCU GearboxOut11 ==
  In : Inport
  BusCreator : BusCreator  Inputs=6
  Demux : Demux  Outputs=6
      settings: DisplayOption=none
  Out : Outport  VectorParamsAs1DForOutWhenUnconnected=off
  wires:
  Demux/6 -> BusCreator/6  "TCU GearboxOut11 Clutch_dis Pos"
  Demux/5 -> BusCreator/5  "TCU GearboxOut11 Clutch Pos"
  Demux/4 -> BusCreator/4  "TCU GearboxOut11 i_trg"
  Demux/3 -> BusCreator/3  "TCU GearboxOut11 set_ParkBrake"
  Demux/2 -> BusCreator/2  "TCU GearboxOut11 GearNoTrg_dis"
  Demux/1 -> BusCreator/1  "TCU GearboxOut11 GearNoTrg"
  BusCreator/1 -> Out/1
  In/1 -> Demux/1

== system PTTransmCU/CarMaker/IPG Vehicle/PowerTrain/TCU Example/PTTransmCU_In/CreateBus TCU GearboxOut2 ==
  In : Inport
  BusCreator : BusCreator  Inputs=6
  Demux : Demux  Outputs=6
      settings: DisplayOption=none
  Out : Outport  VectorParamsAs1DForOutWhenUnconnected=off
  wires:
  Demux/6 -> BusCreator/6  "TCU GearboxOut2 Clutch_dis Pos"
  Demux/5 -> BusCreator/5  "TCU GearboxOut2 Clutch Pos"
  Demux/4 -> BusCreator/4  "TCU GearboxOut2 i_trg"
  Demux/3 -> BusCreator/3  "TCU GearboxOut2 set_ParkBrake"
  Demux/2 -> BusCreator/2  "TCU GearboxOut2 GearNoTrg_dis"
  Demux/1 -> BusCreator/1  "TCU GearboxOut2 GearNoTrg"
  BusCreator/1 -> Out/1
  In/1 -> Demux/1

== system PTTransmCU/CarMaker/IPG Vehicle/PowerTrain/TCU Example/PTTransmCU_In/CreateBus TCU GearboxOut3 ==
  In : Inport
  BusCreator : BusCreator  Inputs=6
  Demux : Demux  Outputs=6
      settings: DisplayOption=none
  Out : Outport  VectorParamsAs1DForOutWhenUnconnected=off
  wires:
  Demux/6 -> BusCreator/6  "TCU GearboxOut3 Clutch_dis Pos"
  Demux/5 -> BusCreator/5  "TCU GearboxOut3 Clutch Pos"
  Demux/4 -> BusCreator/4  "TCU GearboxOut3 i_trg"
  Demux/3 -> BusCreator/3  "TCU GearboxOut3 set_ParkBrake"
  Demux/2 -> BusCreator/2  "TCU GearboxOut3 GearNoTrg_dis"
  Demux/1 -> BusCreator/1  "TCU GearboxOut3 GearNoTrg"
  BusCreator/1 -> Out/1
  In/1 -> Demux/1

== system PTTransmCU/CarMaker/IPG Vehicle/PowerTrain/TCU Example/PTTransmCU_In/CreateBus TCU GearboxOut4 ==
  In : Inport
  BusCreator : BusCreator  Inputs=6
  Demux : Demux  Outputs=6
      settings: DisplayOption=none
  Out : Outport  VectorParamsAs1DForOutWhenUnconnected=off
  wires:
  Demux/6 -> BusCreator/6  "TCU GearboxOut4 Clutch_dis Pos"
  Demux/5 -> BusCreator/5  "TCU GearboxOut4 Clutch Pos"
  Demux/4 -> BusCreator/4  "TCU GearboxOut4 i_trg"
  Demux/3 -> BusCreator/3  "TCU GearboxOut4 set_ParkBrake"
  Demux/2 -> BusCreator/2  "TCU GearboxOut4 GearNoTrg_dis"
  Demux/1 -> BusCreator/1  "TCU GearboxOut4 GearNoTrg"
  BusCreator/1 -> Out/1
  In/1 -> Demux/1

== system PTTransmCU/CarMaker/IPG Vehicle/PowerTrain/TCU Example/PTTransmCU_In/CreateBus TCU GearboxOut5 ==
  In : Inport
  BusCreator : BusCreator  Inputs=6
  Demux : Demux  Outputs=6
      settings: DisplayOption=none
  Out : Outport  VectorParamsAs1DForOutWhenUnconnected=off
  wires:
  Demux/6 -> BusCreator/6  "TCU GearboxOut5 Clutch_dis Pos"
  Demux/5 -> BusCreator/5  "TCU GearboxOut5 Clutch Pos"
  Demux/4 -> BusCreator/4  "TCU GearboxOut5 i_trg"
  Demux/3 -> BusCreator/3  "TCU GearboxOut5 set_ParkBrake"
  Demux/2 -> BusCreator/2  "TCU GearboxOut5 GearNoTrg_dis"
  Demux/1 -> BusCreator/1  "TCU GearboxOut5 GearNoTrg"
  BusCreator/1 -> Out/1
  In/1 -> Demux/1

== system PTTransmCU/CarMaker/IPG Vehicle/PowerTrain/TCU Example/PTTransmCU_In/CreateBus TCU GearboxOut6 ==
  In : Inport
  BusCreator : BusCreator  Inputs=6
  Demux : Demux  Outputs=6
      settings: DisplayOption=none
  Out : Outport  VectorParamsAs1DForOutWhenUnconnected=off
  wires:
  Demux/6 -> BusCreator/6  "TCU GearboxOut6 Clutch_dis Pos"
  Demux/5 -> BusCreator/5  "TCU GearboxOut6 Clutch Pos"
  Demux/4 -> BusCreator/4  "TCU GearboxOut6 i_trg"
  Demux/3 -> BusCreator/3  "TCU GearboxOut6 set_ParkBrake"
  Demux/2 -> BusCreator/2  "TCU GearboxOut6 GearNoTrg_dis"
  Demux/1 -> BusCreator/1  "TCU GearboxOut6 GearNoTrg"
  BusCreator/1 -> Out/1
  In/1 -> Demux/1

== system PTTransmCU/CarMaker/IPG Vehicle/PowerTrain/TCU Example/PTTransmCU_In/CreateBus TCU GearboxOut7 ==
  In : Inport
  BusCreator : BusCreator  Inputs=6
  Demux : Demux  Outputs=6
      settings: DisplayOption=none
  Out : Outport  VectorParamsAs1DForOutWhenUnconnected=off
  wires:
  Demux/6 -> BusCreator/6  "TCU GearboxOut7 Clutch_dis Pos"
  Demux/5 -> BusCreator/5  "TCU GearboxOut7 Clutch Pos"
  Demux/4 -> BusCreator/4  "TCU GearboxOut7 i_trg"
  Demux/3 -> BusCreator/3  "TCU GearboxOut7 set_ParkBrake"
  Demux/2 -> BusCreator/2  "TCU GearboxOut7 GearNoTrg_dis"
  Demux/1 -> BusCreator/1  "TCU GearboxOut7 GearNoTrg"
  BusCreator/1 -> Out/1
  In/1 -> Demux/1

== system PTTransmCU/CarMaker/IPG Vehicle/PowerTrain/TCU Example/PTTransmCU_In/CreateBus TCU GearboxOut8 ==
  In : Inport
  BusCreator : BusCreator  Inputs=6
  Demux : Demux  Outputs=6
      settings: DisplayOption=none
  Out : Outport  VectorParamsAs1DForOutWhenUnconnected=off
  wires:
  Demux/6 -> BusCreator/6  "TCU GearboxOut8 Clutch_dis Pos"
  Demux/5 -> BusCreator/5  "TCU GearboxOut8 Clutch Pos"
  Demux/4 -> BusCreator/4  "TCU GearboxOut8 i_trg"
  Demux/3 -> BusCreator/3  "TCU GearboxOut8 set_ParkBrake"
  Demux/2 -> BusCreator/2  "TCU GearboxOut8 GearNoTrg_dis"
  Demux/1 -> BusCreator/1  "TCU GearboxOut8 GearNoTrg"
  BusCreator/1 -> Out/1
  In/1 -> Demux/1

== system PTTransmCU/CarMaker/IPG Vehicle/PowerTrain/TCU Example/PTTransmCU_In/CreateBus TCU GearboxOut9 ==
  In : Inport
  BusCreator : BusCreator  Inputs=6
  Demux : Demux  Outputs=6
      settings: DisplayOption=none
  Out : Outport  VectorParamsAs1DForOutWhenUnconnected=off
  wires:
  Demux/6 -> BusCreator/6  "TCU GearboxOut9 Clutch_dis Pos"
  Demux/5 -> BusCreator/5  "TCU GearboxOut9 Clutch Pos"
  Demux/4 -> BusCreator/4  "TCU GearboxOut9 i_trg"
  Demux/3 -> BusCreator/3  "TCU GearboxOut9 set_ParkBrake"
  Demux/2 -> BusCreator/2  "TCU GearboxOut9 GearNoTrg_dis"
  Demux/1 -> BusCreator/1  "TCU GearboxOut9 GearNoTrg"
  BusCreator/1 -> Out/1
  In/1 -> Demux/1

== system PTTransmCU/CarMaker/IPG Vehicle/PowerTrain/TCU Example/PTTransmCU_In/CreateBus TCU Input ==
  In : Inport
  BusCreator : BusCreator  Inputs=3
  Demux : Demux  Outputs=3
      settings: DisplayOption=none
  Out : Outport  VectorParamsAs1DForOutWhenUnconnected=off
  wires:
  Demux/3 -> BusCreator/3  "TCU SelectorCtrl"
  Demux/2 -> BusCreator/2  "TCU Load"
  Demux/1 -> BusCreator/1  "TCU Ignition"
  BusCreator/1 -> Out/1
  In/1 -> Demux/1

== system PTTransmCU/CarMaker/IPG Vehicle/PowerTrain/TCU Example/PTTransmCU_In/CreateBus TCU_Cfg Gearbox0 ==
  In : Inport
  BusCreator : BusCreator  Inputs=38
  Demux : Demux  Outputs=38
      settings: DisplayOption=none
  Out : Outport  VectorParamsAs1DForOutWhenUnconnected=off
  wires:
  Demux/38 -> BusCreator/38  "TCU_Cfg Gearbox0 iBGear16"
  Demux/37 -> BusCreator/37  "TCU_Cfg Gearbox0 iBGear15"
  Demux/36 -> BusCreator/36  "TCU_Cfg Gearbox0 iBGear14"
  Demux/35 -> BusCreator/35  "TCU_Cfg Gearbox0 iBGear13"
  Demux/34 -> BusCreator/34  "TCU_Cfg Gearbox0 iBGear12"
  Demux/33 -> BusCreator/33  "TCU_Cfg Gearbox0 iBGear11"
  Demux/32 -> BusCreator/32  "TCU_Cfg Gearbox0 iBGear10"
  Demux/31 -> BusCreator/31  "TCU_Cfg Gearbox0 iBGear9"
  Demux/30 -> BusCreator/30  "TCU_Cfg Gearbox0 iBGear8"
  Demux/29 -> BusCreator/29  "TCU_Cfg Gearbox0 iBGear7"
  Demux/28 -> BusCreator/28  "TCU_Cfg Gearbox0 iBGear6"
  Demux/27 -> BusCreator/27  "TCU_Cfg Gearbox0 iBGear5"
  Demux/26 -> BusCreator/26  "TCU_Cfg Gearbox0 iBGear4"
  Demux/25 -> BusCreator/25  "TCU_Cfg Gearbox0 iBGear3"
  Demux/24 -> BusCreator/24  "TCU_Cfg Gearbox0 iBGear2"
  Demux/23 -> BusCreator/23  "TCU_Cfg Gearbox0 iBGear1"
  Demux/22 -> BusCreator/22  "TCU_Cfg Gearbox0 iBGear0"
  Demux/21 -> BusCreator/21  "TCU_Cfg Gearbox0 nBGears"
  Demux/20 -> BusCreator/20  "TCU_Cfg Gearbox0 iFGear16"
  Demux/19 -> BusCreator/19  "TCU_Cfg Gearbox0 iFGear15"
  Demux/18 -> BusCreator/18  "TCU_Cfg Gearbox0 iFGear14"
  Demux/17 -> BusCreator/17  "TCU_Cfg Gearbox0 iFGear13"
  Demux/16 -> BusCreator/16  "TCU_Cfg Gearbox0 iFGear12"
  Demux/15 -> BusCreator/15  "TCU_Cfg Gearbox0 iFGear11"
  Demux/14 -> BusCreator/14  "TCU_Cfg Gearbox0 iFGear10"
  Demux/13 -> BusCreator/13  "TCU_Cfg Gearbox0 iFGear9"
  Demux/12 -> BusCreator/12  "TCU_Cfg Gearbox0 iFGear8"
  Demux/11 -> BusCreator/11  "TCU_Cfg Gearbox0 iFGear7"
  Demux/10 -> BusCreator/10  "TCU_Cfg Gearbox0 iFGear6"
  Demux/9 -> BusCreator/9  "TCU_Cfg Gearbox0 iFGear5"
  Demux/8 -> BusCreator/8  "TCU_Cfg Gearbox0 iFGear4"
  Demux/7 -> BusCreator/7  "TCU_Cfg Gearbox0 iFGear3"
  Demux/6 -> BusCreator/6  "TCU_Cfg Gearbox0 iFGear2"
  Demux/5 -> BusCreator/5  "TCU_Cfg Gearbox0 iFGear1"
  Demux/4 -> BusCreator/4  "TCU_Cfg Gearbox0 iFGear0"
  Demux/3 -> BusCreator/3  "TCU_Cfg Gearbox0 nFGears"
  Demux/2 -> BusCreator/2  "TCU_Cfg Gearbox0 ClKind"
  Demux/1 -> BusCreator/1  "TCU_Cfg Gearbox0 GBKind"
  BusCreator/1 -> Out/1
  In/1 -> Demux/1

== system PTTransmCU/CarMaker/IPG Vehicle/PowerTrain/TCU Example/PTTransmCU_In/CreateBus TCU_Cfg Gearbox1 ==
  In : Inport
  BusCreator : BusCreator  Inputs=38
  Demux : Demux  Outputs=38
      settings: DisplayOption=none
  Out : Outport  VectorParamsAs1DForOutWhenUnconnected=off
  wires:
  Demux/38 -> BusCreator/38  "TCU_Cfg Gearbox1 iBGear16"
  Demux/37 -> BusCreator/37  "TCU_Cfg Gearbox1 iBGear15"
  Demux/36 -> BusCreator/36  "TCU_Cfg Gearbox1 iBGear14"
  Demux/35 -> BusCreator/35  "TCU_Cfg Gearbox1 iBGear13"
  Demux/34 -> BusCreator/34  "TCU_Cfg Gearbox1 iBGear12"
  Demux/33 -> BusCreator/33  "TCU_Cfg Gearbox1 iBGear11"
  Demux/32 -> BusCreator/32  "TCU_Cfg Gearbox1 iBGear10"
  Demux/31 -> BusCreator/31  "TCU_Cfg Gearbox1 iBGear9"
  Demux/30 -> BusCreator/30  "TCU_Cfg Gearbox1 iBGear8"
  Demux/29 -> BusCreator/29  "TCU_Cfg Gearbox1 iBGear7"
  Demux/28 -> BusCreator/28  "TCU_Cfg Gearbox1 iBGear6"
  Demux/27 -> BusCreator/27  "TCU_Cfg Gearbox1 iBGear5"
  Demux/26 -> BusCreator/26  "TCU_Cfg Gearbox1 iBGear4"
  Demux/25 -> BusCreator/25  "TCU_Cfg Gearbox1 iBGear3"
  Demux/24 -> BusCreator/24  "TCU_Cfg Gearbox1 iBGear2"
  Demux/23 -> BusCreator/23  "TCU_Cfg Gearbox1 iBGear1"
  Demux/22 -> BusCreator/22  "TCU_Cfg Gearbox1 iBGear0"
  Demux/21 -> BusCreator/21  "TCU_Cfg Gearbox1 nBGears"
  Demux/20 -> BusCreator/20  "TCU_Cfg Gearbox1 iFGear16"
  Demux/19 -> BusCreator/19  "TCU_Cfg Gearbox1 iFGear15"
  Demux/18 -> BusCreator/18  "TCU_Cfg Gearbox1 iFGear14"
  Demux/17 -> BusCreator/17  "TCU_Cfg Gearbox1 iFGear13"
  Demux/16 -> BusCreator/16  "TCU_Cfg Gearbox1 iFGear12"
  Demux/15 -> BusCreator/15  "TCU_Cfg Gearbox1 iFGear11"
  Demux/14 -> BusCreator/14  "TCU_Cfg Gearbox1 iFGear10"
  Demux/13 -> BusCreator/13  "TCU_Cfg Gearbox1 iFGear9"
  Demux/12 -> BusCreator/12  "TCU_Cfg Gearbox1 iFGear8"
  Demux/11 -> BusCreator/11  "TCU_Cfg Gearbox1 iFGear7"
  Demux/10 -> BusCreator/10  "TCU_Cfg Gearbox1 iFGear6"
  Demux/9 -> BusCreator/9  "TCU_Cfg Gearbox1 iFGear5"
  Demux/8 -> BusCreator/8  "TCU_Cfg Gearbox1 iFGear4"
  Demux/7 -> BusCreator/7  "TCU_Cfg Gearbox1 iFGear3"
  Demux/6 -> BusCreator/6  "TCU_Cfg Gearbox1 iFGear2"
  Demux/5 -> BusCreator/5  "TCU_Cfg Gearbox1 iFGear1"
  Demux/4 -> BusCreator/4  "TCU_Cfg Gearbox1 iFGear0"
  Demux/3 -> BusCreator/3  "TCU_Cfg Gearbox1 nFGears"
  Demux/2 -> BusCreator/2  "TCU_Cfg Gearbox1 ClKind"
  Demux/1 -> BusCreator/1  "TCU_Cfg Gearbox1 GBKind"
  BusCreator/1 -> Out/1
  In/1 -> Demux/1

== system PTTransmCU/CarMaker/IPG Vehicle/PowerTrain/TCU Example/PTTransmCU_In/CreateBus TCU_Cfg Gearbox10 ==
  In : Inport
  BusCreator : BusCreator  Inputs=38
  Demux : Demux  Outputs=38
      settings: DisplayOption=none
  Out : Outport  VectorParamsAs1DForOutWhenUnconnected=off
  wires:
  Demux/38 -> BusCreator/38  "TCU_Cfg Gearbox10 iBGear16"
  Demux/37 -> BusCreator/37  "TCU_Cfg Gearbox10 iBGear15"
  Demux/36 -> BusCreator/36  "TCU_Cfg Gearbox10 iBGear14"
  Demux/35 -> BusCreator/35  "TCU_Cfg Gearbox10 iBGear13"
  Demux/34 -> BusCreator/34  "TCU_Cfg Gearbox10 iBGear12"
  Demux/33 -> BusCreator/33  "TCU_Cfg Gearbox10 iBGear11"
  Demux/32 -> BusCreator/32  "TCU_Cfg Gearbox10 iBGear10"
  Demux/31 -> BusCreator/31  "TCU_Cfg Gearbox10 iBGear9"
  Demux/30 -> BusCreator/30  "TCU_Cfg Gearbox10 iBGear8"
  Demux/29 -> BusCreator/29  "TCU_Cfg Gearbox10 iBGear7"
  Demux/28 -> BusCreator/28  "TCU_Cfg Gearbox10 iBGear6"
  Demux/27 -> BusCreator/27  "TCU_Cfg Gearbox10 iBGear5"
  Demux/26 -> BusCreator/26  "TCU_Cfg Gearbox10 iBGear4"
  Demux/25 -> BusCreator/25  "TCU_Cfg Gearbox10 iBGear3"
  Demux/24 -> BusCreator/24  "TCU_Cfg Gearbox10 iBGear2"
  Demux/23 -> BusCreator/23  "TCU_Cfg Gearbox10 iBGear1"
  Demux/22 -> BusCreator/22  "TCU_Cfg Gearbox10 iBGear0"
  Demux/21 -> BusCreator/21  "TCU_Cfg Gearbox10 nBGears"
  Demux/20 -> BusCreator/20  "TCU_Cfg Gearbox10 iFGear16"
  Demux/19 -> BusCreator/19  "TCU_Cfg Gearbox10 iFGear15"
  Demux/18 -> BusCreator/18  "TCU_Cfg Gearbox10 iFGear14"
  Demux/17 -> BusCreator/17  "TCU_Cfg Gearbox10 iFGear13"
  Demux/16 -> BusCreator/16  "TCU_Cfg Gearbox10 iFGear12"
  Demux/15 -> BusCreator/15  "TCU_Cfg Gearbox10 iFGear11"
  Demux/14 -> BusCreator/14  "TCU_Cfg Gearbox10 iFGear10"
  Demux/13 -> BusCreator/13  "TCU_Cfg Gearbox10 iFGear9"
  Demux/12 -> BusCreator/12  "TCU_Cfg Gearbox10 iFGear8"
  Demux/11 -> BusCreator/11  "TCU_Cfg Gearbox10 iFGear7"
  Demux/10 -> BusCreator/10  "TCU_Cfg Gearbox10 iFGear6"
  Demux/9 -> BusCreator/9  "TCU_Cfg Gearbox10 iFGear5"
  Demux/8 -> BusCreator/8  "TCU_Cfg Gearbox10 iFGear4"
  Demux/7 -> BusCreator/7  "TCU_Cfg Gearbox10 iFGear3"
  Demux/6 -> BusCreator/6  "TCU_Cfg Gearbox10 iFGear2"
  Demux/5 -> BusCreator/5  "TCU_Cfg Gearbox10 iFGear1"
  Demux/4 -> BusCreator/4  "TCU_Cfg Gearbox10 iFGear0"
  Demux/3 -> BusCreator/3  "TCU_Cfg Gearbox10 nFGears"
  Demux/2 -> BusCreator/2  "TCU_Cfg Gearbox10 ClKind"
  Demux/1 -> BusCreator/1  "TCU_Cfg Gearbox10 GBKind"
  BusCreator/1 -> Out/1
  In/1 -> Demux/1

== system PTTransmCU/CarMaker/IPG Vehicle/PowerTrain/TCU Example/PTTransmCU_In/CreateBus TCU_Cfg Gearbox11 ==
  In : Inport
  BusCreator : BusCreator  Inputs=38
  Demux : Demux  Outputs=38
      settings: DisplayOption=none
  Out : Outport  VectorParamsAs1DForOutWhenUnconnected=off
  wires:
  Demux/38 -> BusCreator/38  "TCU_Cfg Gearbox11 iBGear16"
  Demux/37 -> BusCreator/37  "TCU_Cfg Gearbox11 iBGear15"
  Demux/36 -> BusCreator/36  "TCU_Cfg Gearbox11 iBGear14"
  Demux/35 -> BusCreator/35  "TCU_Cfg Gearbox11 iBGear13"
  Demux/34 -> BusCreator/34  "TCU_Cfg Gearbox11 iBGear12"
  Demux/33 -> BusCreator/33  "TCU_Cfg Gearbox11 iBGear11"
  Demux/32 -> BusCreator/32  "TCU_Cfg Gearbox11 iBGear10"
  Demux/31 -> BusCreator/31  "TCU_Cfg Gearbox11 iBGear9"
  Demux/30 -> BusCreator/30  "TCU_Cfg Gearbox11 iBGear8"
  Demux/29 -> BusCreator/29  "TCU_Cfg Gearbox11 iBGear7"
  Demux/28 -> BusCreator/28  "TCU_Cfg Gearbox11 iBGear6"
  Demux/27 -> BusCreator/27  "TCU_Cfg Gearbox11 iBGear5"
  Demux/26 -> BusCreator/26  "TCU_Cfg Gearbox11 iBGear4"
  Demux/25 -> BusCreator/25  "TCU_Cfg Gearbox11 iBGear3"
  Demux/24 -> BusCreator/24  "TCU_Cfg Gearbox11 iBGear2"
  Demux/23 -> BusCreator/23  "TCU_Cfg Gearbox11 iBGear1"
  Demux/22 -> BusCreator/22  "TCU_Cfg Gearbox11 iBGear0"
  Demux/21 -> BusCreator/21  "TCU_Cfg Gearbox11 nBGears"
  Demux/20 -> BusCreator/20  "TCU_Cfg Gearbox11 iFGear16"
  Demux/19 -> BusCreator/19  "TCU_Cfg Gearbox11 iFGear15"
  Demux/18 -> BusCreator/18  "TCU_Cfg Gearbox11 iFGear14"
  Demux/17 -> BusCreator/17  "TCU_Cfg Gearbox11 iFGear13"
  Demux/16 -> BusCreator/16  "TCU_Cfg Gearbox11 iFGear12"
  Demux/15 -> BusCreator/15  "TCU_Cfg Gearbox11 iFGear11"
  Demux/14 -> BusCreator/14  "TCU_Cfg Gearbox11 iFGear10"
  Demux/13 -> BusCreator/13  "TCU_Cfg Gearbox11 iFGear9"
  Demux/12 -> BusCreator/12  "TCU_Cfg Gearbox11 iFGear8"
  Demux/11 -> BusCreator/11  "TCU_Cfg Gearbox11 iFGear7"
  Demux/10 -> BusCreator/10  "TCU_Cfg Gearbox11 iFGear6"
  Demux/9 -> BusCreator/9  "TCU_Cfg Gearbox11 iFGear5"
  Demux/8 -> BusCreator/8  "TCU_Cfg Gearbox11 iFGear4"
  Demux/7 -> BusCreator/7  "TCU_Cfg Gearbox11 iFGear3"
  Demux/6 -> BusCreator/6  "TCU_Cfg Gearbox11 iFGear2"
  Demux/5 -> BusCreator/5  "TCU_Cfg Gearbox11 iFGear1"
  Demux/4 -> BusCreator/4  "TCU_Cfg Gearbox11 iFGear0"
  Demux/3 -> BusCreator/3  "TCU_Cfg Gearbox11 nFGears"
  Demux/2 -> BusCreator/2  "TCU_Cfg Gearbox11 ClKind"
  Demux/1 -> BusCreator/1  "TCU_Cfg Gearbox11 GBKind"
  BusCreator/1 -> Out/1
  In/1 -> Demux/1

== system PTTransmCU/CarMaker/IPG Vehicle/PowerTrain/TCU Example/PTTransmCU_In/CreateBus TCU_Cfg Gearbox2 ==
  In : Inport
  BusCreator : BusCreator  Inputs=38
  Demux : Demux  Outputs=38
      settings: DisplayOption=none
  Out : Outport  VectorParamsAs1DForOutWhenUnconnected=off
  wires:
  Demux/38 -> BusCreator/38  "TCU_Cfg Gearbox2 iBGear16"
  Demux/37 -> BusCreator/37  "TCU_Cfg Gearbox2 iBGear15"
  Demux/36 -> BusCreator/36  "TCU_Cfg Gearbox2 iBGear14"
  Demux/35 -> BusCreator/35  "TCU_Cfg Gearbox2 iBGear13"
  Demux/34 -> BusCreator/34  "TCU_Cfg Gearbox2 iBGear12"
  Demux/33 -> BusCreator/33  "TCU_Cfg Gearbox2 iBGear11"
  Demux/32 -> BusCreator/32  "TCU_Cfg Gearbox2 iBGear10"
  Demux/31 -> BusCreator/31  "TCU_Cfg Gearbox2 iBGear9"
  Demux/30 -> BusCreator/30  "TCU_Cfg Gearbox2 iBGear8"
  Demux/29 -> BusCreator/29  "TCU_Cfg Gearbox2 iBGear7"
  Demux/28 -> BusCreator/28  "TCU_Cfg Gearbox2 iBGear6"
  Demux/27 -> BusCreator/27  "TCU_Cfg Gearbox2 iBGear5"
  Demux/26 -> BusCreator/26  "TCU_Cfg Gearbox2 iBGear4"
  Demux/25 -> BusCreator/25  "TCU_Cfg Gearbox2 iBGear3"
  Demux/24 -> BusCreator/24  "TCU_Cfg Gearbox2 iBGear2"
  Demux/23 -> BusCreator/23  "TCU_Cfg Gearbox2 iBGear1"
  Demux/22 -> BusCreator/22  "TCU_Cfg Gearbox2 iBGear0"
  Demux/21 -> BusCreator/21  "TCU_Cfg Gearbox2 nBGears"
  Demux/20 -> BusCreator/20  "TCU_Cfg Gearbox2 iFGear16"
  Demux/19 -> BusCreator/19  "TCU_Cfg Gearbox2 iFGear15"
  Demux/18 -> BusCreator/18  "TCU_Cfg Gearbox2 iFGear14"
  Demux/17 -> BusCreator/17  "TCU_Cfg Gearbox2 iFGear13"
  Demux/16 -> BusCreator/16  "TCU_Cfg Gearbox2 iFGear12"
  Demux/15 -> BusCreator/15  "TCU_Cfg Gearbox2 iFGear11"
  Demux/14 -> BusCreator/14  "TCU_Cfg Gearbox2 iFGear10"
  Demux/13 -> BusCreator/13  "TCU_Cfg Gearbox2 iFGear9"
  Demux/12 -> BusCreator/12  "TCU_Cfg Gearbox2 iFGear8"
  Demux/11 -> BusCreator/11  "TCU_Cfg Gearbox2 iFGear7"
  Demux/10 -> BusCreator/10  "TCU_Cfg Gearbox2 iFGear6"
  Demux/9 -> BusCreator/9  "TCU_Cfg Gearbox2 iFGear5"
  Demux/8 -> BusCreator/8  "TCU_Cfg Gearbox2 iFGear4"
  Demux/7 -> BusCreator/7  "TCU_Cfg Gearbox2 iFGear3"
  Demux/6 -> BusCreator/6  "TCU_Cfg Gearbox2 iFGear2"
  Demux/5 -> BusCreator/5  "TCU_Cfg Gearbox2 iFGear1"
  Demux/4 -> BusCreator/4  "TCU_Cfg Gearbox2 iFGear0"
  Demux/3 -> BusCreator/3  "TCU_Cfg Gearbox2 nFGears"
  Demux/2 -> BusCreator/2  "TCU_Cfg Gearbox2 ClKind"
  Demux/1 -> BusCreator/1  "TCU_Cfg Gearbox2 GBKind"
  BusCreator/1 -> Out/1
  In/1 -> Demux/1
